simulink library "aerolibguid"  (Simulink 5.0)
libraries: simulink x1
settings Model: Creator=sgage  LastModifiedBy=sgage  ExtModeAutoUpdateStatusClock=off  TargetHWChar=2  TargetHWWordLengths=8,16,32,32

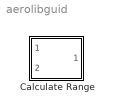
== system aerolibguid ==
  Calculate Range : Subsystem
      mask Type: Calculate Range
      mask Description: Calculate range between craft 2 and craft 1 given their respective positions. Range is always positive.
      mask Help: web(asbhelp);
      mask Display:
      | port_label('input',1,'X_1','texmode','on');
      | port_label('input',2,'X_2','texmode','on');
      | port_label('output',1,'R_{2-1}','texmode','on');

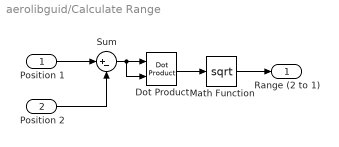
== system aerolibguid/Calculate Range ==
  Position 1 : Inport  ShowAdditionalParam=on
  Position 2 : Inport  Port=2  ShowAdditionalParam=on
  Dot Product : simulink/Math Operations/Dot Product
  Math Function : Math  Operator=sqrt
  Sum : Sum  Inputs=|+-  SaturateOnIntegerOverflow=on
  Range (2 to 1) : Outport
  wires:
  Sum/1 -> Dot Product/2, Dot Product/1
  Dot Product/1 -> Math Function/1
  Position 2/1 -> Sum/2
  Position 1/1 -> Sum/1
  Math Function/1 -> Range (2 to 1)/1
